simulink model "three_level_ttype_pwm"  (R2025a)
settings: Solver=ode1be  StartTime=0.0  StopTime=simlength  FixedStep=ts_sim  MaxStep=ts_sim
undefined symbols (not defined in the file): fPWM_INV, kp_dudc, number_of_cells, Q, q1Kalman, q2Kalman, q3Kalman, rKalman, tc, ts_zvs, tsample, Vbattery_nom
libraries: fl_lib x54, nesl_utility x31, lithium_ion_cell_lib x1, simulink x1
(part 1 of 2)
settings Model: SimulationMode=accelerator  Creator=LTNBDA  LastModifiedBy=ltnbda
settings SolverCC: ZeroCrossControl=EnableAll  ZeroCrossAlgorithm=Adaptive  AlgebraicLoopSolver=TrustRegion  SolverResetMethod=Robust  AutoInsertRateTranBlk=on
settings DataIOCC: LimitDataPoints=on  MaxDataPoints=1  SaveFormat=Array  SignalLoggingSaveFormat=ModelDataLogs  SaveOutput=off  SignalLogging=off  DSMLogging=off  SaveTime=off  ReturnWorkspaceOutputs=off
settings OptimizationCC: ExpressionDepthLimit=2147483647.0  InitFltsAndDblsToZero=on  EfficientMapNaN2IntZero=off  LifeSpan=inf
settings DebuggingCC: SaveWithParameterizedLinksMsg=none  UnderspecifiedInitializationDetection=Classic  MergeDetectMultiDrivingBlocksExec=none  SignalResolutionControl=TryResolveAllWithWarning  SolverPrmCheckMsg=warning  MultiTaskDSMMsg=warning  MultiTaskCondExecSysMsg=none  MultiTaskRateTransMsg=warning  FcnCallInpInsideContextMsg=warning  StateNameClashWarn=warning  SFUnexpectedBacktrackingDiag=warning  SFNoUnconditionalDefaultTransitionDiag=warning  ArithmeticOperatorsInVariantConditions=warning
settings HardwareCC: ProdBitPerLong=64.0  ProdLargestAtomicFloat=None  ProdIntDivRoundTo=Undefined  ProdEndianess=Unspecified  ProdHWDeviceType=Generic->64-bit Embedded Processor (LP64)  TargetBitPerPointer=64.0  TargetBitPerSizeT=64.0  TargetBitPerPtrDiffT=64.0  TargetLongLongMode=on  TargetIntDivRoundTo=Zero  TargetEndianess=LittleEndian  TargetWordSize=64.0  TargetHWDeviceType=MATLAB Host  ProdEqTarget=off
settings ModelReferenceCC: EnableRefExpFcnMdlSchedulingChecks=on  PropagateSignalLabelsOutOfModel=off
settings SFSimCC: SimUseLocalCustomCode=off  CustomCodeUndefinedFunction=UseInterfaceOnly
settings RTWCC: RTWUseLocalCustomCode=off  GPUComputeCapability=3.5
settings CodeAppCC: MaxIdLength=128.0  StateflowObjectComments=on
settings GRTTargetCC: TargetLangStandard=C89/C90 (ANSI)  CombineOutputUpdateFcns=off  GRTInterface=on
settings ConfigComp: CovMetricSettings=dw  CovSaveCumulativeToWorkspaceVar=on  CovSaveSingleToWorkspaceVar=on  CovExternalEMLEnable=off
settings SimscapeCC: SimscapeNormalizeSystem=off

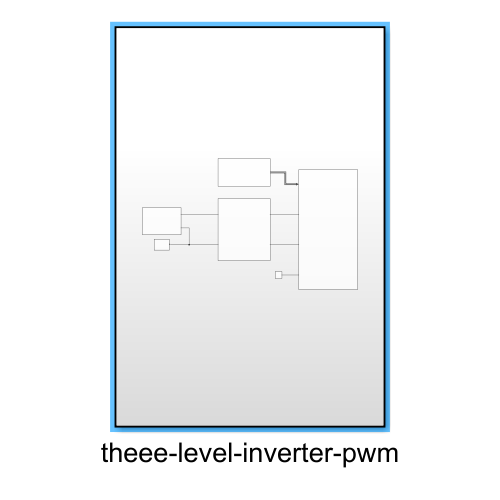
[thumbnail: Simulink's stored preview of the top-level diagram]
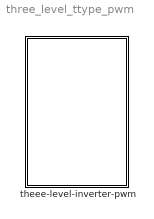
== system three_level_ttype_pwm ==
  theee-level-inverter-pwm : Subsystem

== system three_level_ttype_pwm/theee-level-inverter-pwm ==
  Electrical Reference2 : fl_lib/Electrical/Electrical Elements/Electrical Reference
  Solver Configuration : nesl_utility/Solver Configuration  PhysicalDomain=network_engine_domain  SubClassName=solver  LeftPortType=input  RightPortType=generic  Tones=[]  Harmonics=[]  SimulateNoise=off  Profile=off  UseLocalSampling=off  EnableSwitchedLinearOptims=on  FrequencyDomain=off  UseCCode=off  RelTol=0.001  AbsTol=0.001  MinStep=1e-09  ToWorkspace=off  RevertToSquareIcSolve=off  NumHomotopyIterations=100  PhasorMode=off  PhasorModeNumHarmonics=1  ConsistencySolver=NEWTON_FTOL  IndexReductionMethod=DerivativeReplacement  DoDC=on  ResidualTolerance=1e-09  ConsistencyTolSource=GLOBAL  ConsistencyAbsTol=0.001  ConsistencyRelTol=0.001  ConsistencyTolFactor=0.001  UseLocalSolver=on  LocalSolverChoice=NE_BACKWARD_EULER_ADVANCER  ResolveIndetEquations=on  FunctionEvalNumThread=1  LocalSolverSampleTime=ts_sim  DoFixedCost=off  MaxNonlinIter=3  MaxModeIter=2  ComputeImpulses=off  ImpulseIterations=2  LinearAlgebra=auto  LinearAlgebraNumThread=0  EquationFormulation=NE_TIME_EF  DelaysMemoryBudget=1024  AutomaticFiltering=on  FilteringTimeConstant=0.001  PartitionStorageMethod=AS_NEEDED  PartitionMemoryBudget=1024  PartitionMethod=ROBUST  MultibodyUseLocalSolver=off  MultibodyLocalSolverChoice=ODE1  MultibodyLocalSolverSampleTime=0.001
  battery_system : Subsystem
  pwm_commands : Subsystem
  single_phase_ui_measure1 : Subsystem
  three-level-inverter : Subsystem
  wires:
  pwm_commands/1(gate_commands) -> three-level-inverter/1(gate_commands)
  connections:
  single_phase_ui_measure1/LConn2 -- Solver Configuration/RConn1 -- battery_system/RConn2
  single_phase_ui_measure1/RConn1 -- three-level-inverter/LConn1
  battery_system/RConn1 -- single_phase_ui_measure1/LConn1
  three-level-inverter/LConn2 -- single_phase_ui_measure1/RConn2
  Electrical Reference2/LConn1 -- three-level-inverter/LConn3

== system three_level_ttype_pwm/theee-level-inverter-pwm/battery_system ==
  LithiumIonBattery : Subsystem
  Uout+ : PMIOPort  Side=Right
  Uout- : PMIOPort  Port=2  Side=Right
  connections:
  LithiumIonBattery/RConn1 -- Uout+/RConn1
  LithiumIonBattery/RConn2 -- Uout-/RConn1

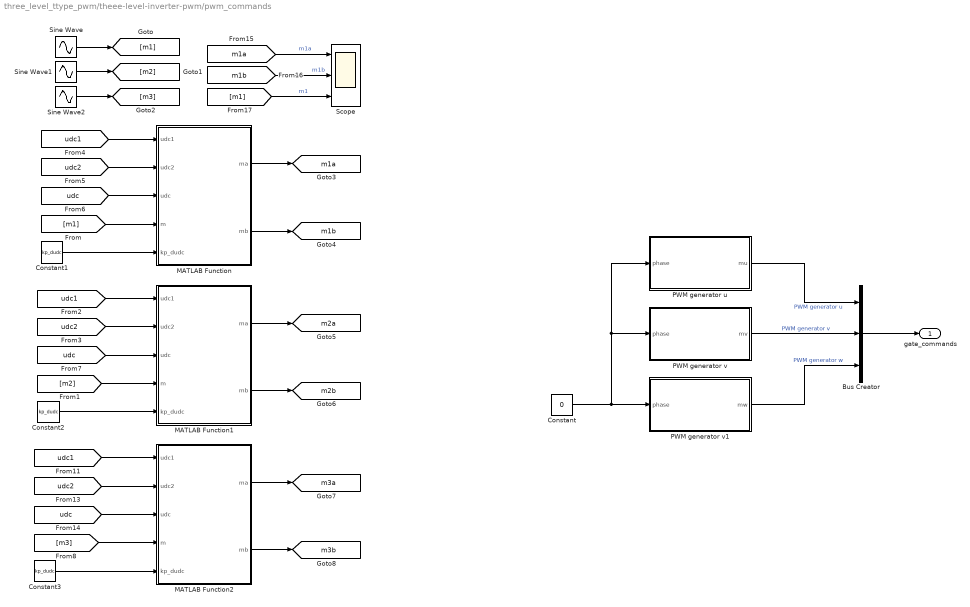
== system three_level_ttype_pwm/theee-level-inverter-pwm/pwm_commands ==
  Bus Creator : BusCreator  Inputs=3
  Constant : Constant  Value=0
  Constant1 : Constant  Value=kp_dudc
  Constant2 : Constant  Value=kp_dudc
  Constant3 : Constant  Value=kp_dudc
  MATLAB Function : MATLAB Function  TreatAsAtomicUnit=on
  MATLAB Function1 : MATLAB Function  TreatAsAtomicUnit=on
  MATLAB Function2 : MATLAB Function  TreatAsAtomicUnit=on
  PWM generator u : Subsystem  mask{f=fPWM_INV, m_up=1, m_low=-1, dead_time=0, pos_cmd_gate=1, neg_cmd_gate=0, polarity=1}
      mask prompts: f "Frequency (Hz)"; m_up "Max Input Modulation Value"; m_low "Min Input Modulation Value"; dead_time "Dead Time (s)"; pos_cmd_gate "Positive Gate Voltage (V)"; neg_cmd_gate "Negative Gate Voltage (V)"; polarity "Polarity (pu)"
  PWM generator v : Subsystem  mask{f=fPWM_INV, m_up=1, m_low=-1, dead_time=0, pos_cmd_gate=1, neg_cmd_gate=0, polarity=1}
      mask prompts: f "Frequency (Hz)"; m_up "Max Input Modulation Value"; m_low "Min Input Modulation Value"; dead_time "Dead Time (s)"; pos_cmd_gate "Positive Gate Voltage (V)"; neg_cmd_gate "Negative Gate Voltage (V)"; polarity "Polarity (pu)"
  PWM generator v1 : Subsystem  mask{f=fPWM_INV, m_up=1, m_low=-1, dead_time=0, pos_cmd_gate=1, neg_cmd_gate=0, polarity=1}
      mask prompts: f "Frequency (Hz)"; m_up "Max Input Modulation Value"; m_low "Min Input Modulation Value"; dead_time "Dead Time (s)"; pos_cmd_gate "Positive Gate Voltage (V)"; neg_cmd_gate "Negative Gate Voltage (V)"; polarity "Polarity (pu)"
  Scope : Scope  NumInputPorts=3
      settings: ActiveDisplayYMinimum=-1.0203710782461322  ActiveDisplayYMaximum=1.0167997732254843
  Sine Wave : Sin  Amplitude=0.8  Frequency=2*pi*50  SampleTime=0
  Sine Wave1 : Sin  Amplitude=0.8  Frequency=2*pi*50  Phase=-2*pi/3  SampleTime=0
  Sine Wave2 : Sin  Amplitude=0.8  Frequency=2*pi*50  Phase=2*pi/3  SampleTime=0
  gate_commands : Outport
  tag scope: m1a=global, m1b=global, m2a=global, m2b=global, m3a=global, m3b=global
  wires:
  PWM generator v/1(mv) -> Bus Creator/2  "PWM generator v"
  PWM generator u/1(mu) -> Bus Creator/1  "PWM generator u"
  PWM generator v1/1(mw) -> Bus Creator/3  "PWM generator w"
  Constant/1 -> PWM generator u/1(phase), PWM generator v/1(phase), PWM generator v1/1(phase)
  Sine Wave/1 -> [m1]
  Sine Wave1/1 -> [m2]
  Sine Wave2/1 -> [m3]
  [m1] -> MATLAB Function/4(m)
  MATLAB Function/1(ma) -> [m1a]
  MATLAB Function/2(mb) -> [m1b]
  MATLAB Function1/1(ma) -> [m2a]
  MATLAB Function1/2(mb) -> [m2b]
  [m2] -> MATLAB Function1/4(m)
  MATLAB Function2/1(ma) -> [m3a]
  MATLAB Function2/2(mb) -> [m3b]
  [m1a] -> Scope/1  "m1a"
  [m1b] -> Scope/2  "m1b"
  [m3] -> MATLAB Function2/4(m)
  [udc] -> MATLAB Function/3(udc)
  [udc] -> MATLAB Function1/3(udc)
  [m1] -> Scope/3  "m1"
  [udc] -> MATLAB Function2/3(udc)
  Constant1/1 -> MATLAB Function/5(kp_dudc)
  Constant2/1 -> MATLAB Function1/5(kp_dudc)
  Constant3/1 -> MATLAB Function2/5(kp_dudc)
  [udc1] -> MATLAB Function/1(udc1)
  [udc2] -> MATLAB Function/2(udc2)
  [udc1] -> MATLAB Function1/1(udc1)
  [udc2] -> MATLAB Function1/2(udc2)
  [udc1] -> MATLAB Function2/1(udc1)
  [udc2] -> MATLAB Function2/2(udc2)
  Bus Creator/1 -> gate_commands/1

== system three_level_ttype_pwm/theee-level-inverter-pwm/single_phase_ui_measure1 ==
  Bus Creator : BusCreator  Inputs=2
  Current Sensor : fl_lib/Electrical/Electrical Sensors/Current Sensor
  Selector : Selector  InputPortWidth=2  IndexOptions=Index vector (dialog)  Indices=2  OutputSizes=1
  Selector1 : Selector  InputPortWidth=2  IndexOptions=Index vector (dialog)  Indices=1  OutputSizes=1
  Transfer Fcn : TransferFcn  Denominator=[1e-4 1]
  Voltage Sensor : fl_lib/Electrical/Electrical Sensors/Voltage Sensor
  input : Scope  NumInputPorts=2
      settings: SampleTime=tc  ActiveDisplayYMinimum=-52.828591960664284  ActiveDisplayYMaximum=475.45762649280624  DataLoggingVariableName=ScopeData2
  iph : nesl_utility/PS-Simulink Converter  PhysicalDomain=network_engine_domain  SubClassName=ps_output  LeftPortType=input  RightPortType=output  PseudoPeriodic=off  Frequencies=[]  VectorFormat=1-D array  Unit=A  AffineConversion=off
  uph : nesl_utility/PS-Simulink Converter  PhysicalDomain=network_engine_domain  SubClassName=ps_output  LeftPortType=input  RightPortType=output  PseudoPeriodic=off  Frequencies=[]  VectorFormat=1-D array  Unit=V  AffineConversion=off
  Udc(+) : PMIOPort  Side=Left
  udc(+) : PMIOPort  Port=2  Side=Right
  Udc(-) : PMIOPort  Port=3  Side=Left
  udc(-) : PMIOPort  Port=4  Side=Right
  tag scope: current_battery=global, voltage_battery=global
  wires:
  Selector/1 -> input/2, [voltage_battery]  "voltage_battery"
  Selector1/1 -> input/1, Transfer Fcn/1  "current_battery"
  uph/1 -> Bus Creator/2  "uph"
  iph/1 -> Bus Creator/1  "iph"
  Bus Creator/1 -> Selector1/1, Selector/1  "ui_data"
  Transfer Fcn/1 -> [current_battery]
  connections:
  udc(-)/RConn1 -- Udc(-)/RConn1 -- Voltage Sensor/RConn2
  Voltage Sensor/RConn1 -- uph/LConn1
  Current Sensor/RConn2 -- udc(+)/RConn1
  Udc(+)/RConn1 -- Current Sensor/LConn1 -- Voltage Sensor/LConn1
  iph/LConn1 -- Current Sensor/RConn1

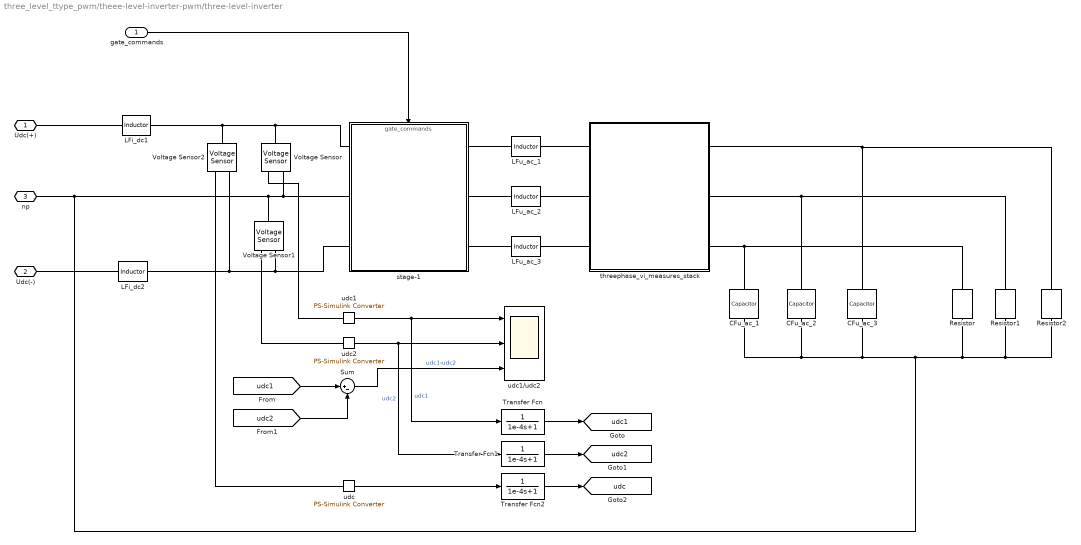
== system three_level_ttype_pwm/theee-level-inverter-pwm/three-level-inverter ==
  gate_commands : Inport
  CFu_ac_1 : fl_lib/Electrical/Electrical Elements/Capacitor  c=400e-6 F  r=5e-3 Ohm  g=0 1/Ohm  i_specify=off  i_priority=None  i=0 A  i_nominal_specify=off  i_nominal_value=1  i_nominal_unit=A  v_specify=off  v_priority=None  v=0 V  v_nominal_specify=off  v_nominal_value=1  v_nominal_unit=V  vc_specify=off  vc_priority=High  vc=0 V  vc_nominal_specify=off  vc_nominal_value=1  vc_nominal_unit=V
  CFu_ac_2 : fl_lib/Electrical/Electrical Elements/Capacitor  c=400e-6 F  r=5e-3 Ohm  g=0 1/Ohm  i_specify=off  i_priority=None  i=0 A  i_nominal_specify=off  i_nominal_value=1  i_nominal_unit=A  v_specify=off  v_priority=None  v=0 V  v_nominal_specify=off  v_nominal_value=1  v_nominal_unit=V  vc_specify=off  vc_priority=High  vc=0 V  vc_nominal_specify=off  vc_nominal_value=1  vc_nominal_unit=V
  CFu_ac_3 : fl_lib/Electrical/Electrical Elements/Capacitor  c=400e-6 F  r=5e-3 Ohm  g=0 1/Ohm  i_specify=off  i_priority=None  i=0 A  i_nominal_specify=off  i_nominal_value=1  i_nominal_unit=A  v_specify=off  v_priority=None  v=0 V  v_nominal_specify=off  v_nominal_value=1  v_nominal_unit=V  vc_specify=off  vc_priority=High  vc=0 V  vc_nominal_specify=off  vc_nominal_value=1  vc_nominal_unit=V
  LFi_dc1 : fl_lib/Electrical/Electrical Elements/Inductor  l=Ldc1 H  r=RLdc1 Ohm  g=1e-9 1/Ohm  i_specify=on  i_priority=High  i=0 A  i_nominal_specify=off  i_nominal_value=1  i_nominal_unit=A  v_specify=off  v_priority=None  v=0 V  v_nominal_specify=off  v_nominal_value=1  v_nominal_unit=V  i_L_specify=off  i_L_priority=High  i_L=0 A  i_L_nominal_specify=off  i_L_nominal_value=1  i_L_nominal_unit=A
  LFi_dc2 : fl_lib/Electrical/Electrical Elements/Inductor  l=Ldc2 H  r=Ldc2 Ohm  g=1e-9 1/Ohm  i_specify=on  i_priority=High  i=0 A  i_nominal_specify=off  i_nominal_value=1  i_nominal_unit=A  v_specify=off  v_priority=None  v=0 V  v_nominal_specify=off  v_nominal_value=1  v_nominal_unit=V  i_L_specify=off  i_L_priority=High  i_L=0 A  i_L_nominal_specify=off  i_L_nominal_value=1  i_L_nominal_unit=A
  LFu_ac_1 : fl_lib/Electrical/Electrical Elements/Inductor  l=250e-6 H  r=3e-3 Ohm  g=1e-9 1/Ohm  i_specify=off  i_priority=None  i=0 A  i_nominal_specify=off  i_nominal_value=1  i_nominal_unit=A  v_specify=off  v_priority=None  v=0 V  v_nominal_specify=off  v_nominal_value=1  v_nominal_unit=V  i_L_specify=off  i_L_priority=High  i_L=0 A  i_L_nominal_specify=off  i_L_nominal_value=1  i_L_nominal_unit=A
  LFu_ac_2 : fl_lib/Electrical/Electrical Elements/Inductor  l=250e-6 H  r=3e-3 Ohm  g=1e-9 1/Ohm  i_specify=off  i_priority=None  i=0 A  i_nominal_specify=off  i_nominal_value=1  i_nominal_unit=A  v_specify=off  v_priority=None  v=0 V  v_nominal_specify=off  v_nominal_value=1  v_nominal_unit=V  i_L_specify=off  i_L_priority=High  i_L=0 A  i_L_nominal_specify=off  i_L_nominal_value=1  i_L_nominal_unit=A
  LFu_ac_3 : fl_lib/Electrical/Electrical Elements/Inductor  l=250e-6 H  r=3e-3 Ohm  g=1e-9 1/Ohm  i_specify=off  i_priority=None  i=0 A  i_nominal_specify=off  i_nominal_value=1  i_nominal_unit=A  v_specify=off  v_priority=None  v=0 V  v_nominal_specify=off  v_nominal_value=1  v_nominal_unit=V  i_L_specify=off  i_L_priority=High  i_L=0 A  i_L_nominal_specify=off  i_L_nominal_value=1  i_L_nominal_unit=A
  Resistor : fl_lib/Electrical/Electrical Elements/Resistor  R=1.6 Ohm  i_specify=off  i_priority=None  i=0 A  i_nominal_specify=off  i_nominal_value=1  i_nominal_unit=A  v_specify=off  v_priority=None  v=0 V  v_nominal_specify=off  v_nominal_value=1  v_nominal_unit=V
  Resistor1 : fl_lib/Electrical/Electrical Elements/Resistor  R=1.6 Ohm  i_specify=off  i_priority=None  i=0 A  i_nominal_specify=off  i_nominal_value=1  i_nominal_unit=A  v_specify=off  v_priority=None  v=0 V  v_nominal_specify=off  v_nominal_value=1  v_nominal_unit=V
  Resistor2 : fl_lib/Electrical/Electrical Elements/Resistor  R=1.6 Ohm  i_specify=off  i_priority=None  i=0 A  i_nominal_specify=off  i_nominal_value=1  i_nominal_unit=A  v_specify=off  v_priority=None  v=0 V  v_nominal_specify=off  v_nominal_value=1  v_nominal_unit=V
  Sum : Sum  Inputs=|+-
  Transfer Fcn : TransferFcn  Denominator=[1e-4 1]
  Transfer Fcn1 : TransferFcn  Denominator=[1e-4 1]
  Transfer Fcn2 : TransferFcn  Denominator=[1e-4 1]
  Voltage Sensor : fl_lib/Electrical/Electrical Sensors/Voltage Sensor
  Voltage Sensor1 : fl_lib/Electrical/Electrical Sensors/Voltage Sensor
  Voltage Sensor2 : fl_lib/Electrical/Electrical Sensors/Voltage Sensor
  stage-1 : Subsystem
      settings: PortSchema="{\"entries\":[{\"content\":{\"sides\":[{\"content\":{\"connectorIds\":[\"LConn1\",\"LConn2\",\"LConn3\"]},\"type\":\"ConnectorPlacement.EquallySpacedRectSide\",\"uuid\":\"c872503a-61af-4937-bdf2-4de4f8645573\"},{\"content\":{\"connectorIds\":[\"RConn1\",\"RConn2\",\"RConn3\"],\"side\":\"RIGHT\"},\"type\":\"ConnectorPlacement.EquallySpacedRectSide\",\"uuid\":\"3b83f060-86a2-4569-84b5-d9f7c0485347\"},{\"content\":{\"connectorIds\":[\"In1\"],\"side\":\"TOP\"},\"type\":\"ConnectorPlacement.EquallySpacedRectSide\",\"uuid\":\"bf191d46-ce71-4d15-9dd0-24cc57253577\"}]},\"type\":\"ConnectorPlacement.EquallySpacedConnector\",\"uuid\":\"1b28ceee-25d0-45ae-a3c4-c2563f0d63ba\"}],\"packageUris\":[\"http://schema.mathworks.com/mf0/Connector/R2020b\"],\"version\":\"1.0\"}"
  threephase_vi_measures_stack : Subsystem
  udc : nesl_utility/PS-Simulink Converter  PhysicalDomain=network_engine_domain  SubClassName=ps_output  LeftPortType=input  RightPortType=output  PseudoPeriodic=off  Frequencies=[]  VectorFormat=1-D array  Unit=V  AffineConversion=off
  udc1 : nesl_utility/PS-Simulink Converter  PhysicalDomain=network_engine_domain  SubClassName=ps_output  LeftPortType=input  RightPortType=output  PseudoPeriodic=off  Frequencies=[]  VectorFormat=1-D array  Unit=V  AffineConversion=off
  udc1/udc2 : Scope  NumInputPorts=3
      settings: SampleTime=tc  ActiveDisplayYMinimum=459.3584684150768  ActiveDisplayYMaximum=553.49695314359838  DataLoggingVariableName=ScopeData5
  udc2 : nesl_utility/PS-Simulink Converter  PhysicalDomain=network_engine_domain  SubClassName=ps_output  LeftPortType=input  RightPortType=output  PseudoPeriodic=off  Frequencies=[]  VectorFormat=1-D array  Unit=V  AffineConversion=off
  Udc(+) : PMIOPort  Side=Left
  Udc(-) : PMIOPort  Port=2  Side=Left
  np : PMIOPort  Port=3  Side=Left
  tag scope: udc1=global, udc2=global, udc=global
  wires:
  udc2/1 -> Transfer Fcn1/1, udc1/udc2/2  "udc2"
  udc1/1 -> Transfer Fcn/1, udc1/udc2/1  "udc1"
  gate_commands/1 -> stage-1/1(gate_commands)
  udc/1 -> Transfer Fcn2/1
  Transfer Fcn/1 -> [udc1]
  Transfer Fcn1/1 -> [udc2]
  Transfer Fcn2/1 -> [udc]
  [udc1] -> Sum/1
  [udc2] -> Sum/2
  Sum/1 -> udc1/udc2/3  "udc1-udc2"
  connections:
  LFi_dc2/RConn1 -- Voltage Sensor2/RConn2 -- stage-1/RConn3 -- Voltage Sensor1/RConn2
  Voltage Sensor/RConn1 -- udc1/LConn1
  Voltage Sensor1/RConn1 -- udc2/LConn1
  CFu_ac_3/LConn1 -- Resistor2/LConn1 -- threephase_vi_measures_stack/RConn1
  CFu_ac_2/LConn1 -- Resistor1/LConn1 -- threephase_vi_measures_stack/RConn2
  threephase_vi_measures_stack/RConn3 -- Resistor/LConn1 -- CFu_ac_1/LConn1
  LFu_ac_3/RConn1 -- threephase_vi_measures_stack/LConn3
  LFu_ac_2/RConn1 -- threephase_vi_measures_stack/LConn2
  LFu_ac_1/RConn1 -- threephase_vi_measures_stack/LConn1
  stage-1/LConn3 -- LFu_ac_3/LConn1
  stage-1/LConn1 -- LFu_ac_1/LConn1
  LFu_ac_2/LConn1 -- stage-1/LConn2
  Voltage Sensor/LConn1 -- LFi_dc1/RConn1 -- Voltage Sensor2/LConn1 -- stage-1/RConn1
  LFi_dc1/LConn1 -- Udc(+)/RConn1
  Voltage Sensor2/RConn1 -- udc/LConn1
  Udc(-)/RConn1 -- LFi_dc2/LConn1
  Voltage Sensor/RConn2 -- np/RConn1 -- Resistor1/RConn1 -- Resistor2/RConn1 -- Resistor/RConn1 -- CFu_ac_2/RConn1 -- CFu_ac_1/RConn1 -- CFu_ac_3/RConn1 -- Voltage Sensor1/LConn1 -- stage-1/RConn2

== system three_level_ttype_pwm/theee-level-inverter-pwm/battery_system/LithiumIonBattery ==
  Current Sensor : fl_lib/Electrical/Electrical Sensors/Current Sensor
  PS-Simulink Converter4 : nesl_utility/PS-Simulink Converter  PhysicalDomain=network_engine_domain  SubClassName=ps_output  LeftPortType=input  RightPortType=output  PseudoPeriodic=off  Frequencies=[]  VectorFormat=1-D array  Unit=1  AffineConversion=off
  PS-Simulink Converter5 : nesl_utility/PS-Simulink Converter  PhysicalDomain=network_engine_domain  SubClassName=ps_output  LeftPortType=input  RightPortType=output  PseudoPeriodic=off  Frequencies=[]  VectorFormat=1-D array  Unit=V  AffineConversion=on
  SOC_estimator : Subsystem  Commented=on
  To Workspace1 : ToWorkspace  VariableName=idc_battery_sim  SampleTime=tc
      settings: MaxDataPoints=Nc
  To Workspace2 : ToWorkspace  VariableName=udc_battery_sim  SampleTime=tc
      settings: MaxDataPoints=Nc
  Unit Delay5 : UnitDelay  SampleTime=ts_zvs  HasFrameUpgradeWarning=on
  Voltage Sensor : fl_lib/Electrical/Electrical Sensors/Voltage Sensor
  ibat/vdc : Scope  NumInputPorts=2
      settings: SampleTime=tc  ActiveDisplayYMinimum=-124.51886598951859  ActiveDisplayYMaximum=1120.6697939056676  DataLoggingVariableName=ScopeData6
  lithium ion cell analytical ocv : Subsystem
  Uout+ : PMIOPort  Side=Right
  Uout- : PMIOPort  Port=2  Side=Right
  wires:
  [vdc] -> ibat/vdc/2  "vdc"
  Unit Delay5/1 -> [vdc], To Workspace2/1
  PS-Simulink Converter4/1 -> ibat/vdc/1, To Workspace1/1  "i batt"
  PS-Simulink Converter5/1 -> Unit Delay5/1
  connections:
  lithium ion cell analytical ocv/RConn1 -- Current Sensor/LConn1
  Uout-/RConn1 -- lithium ion cell analytical ocv/RConn2 -- Voltage Sensor/RConn2
  Voltage Sensor/RConn1 -- PS-Simulink Converter5/LConn1
  Voltage Sensor/LConn1 -- Current Sensor/RConn2 -- Uout+/RConn1
  Current Sensor/RConn1 -- PS-Simulink Converter4/LConn1

== system three_level_ttype_pwm/theee-level-inverter-pwm/pwm_commands/PWM generator u ==
  phase : Inport
  Bus Creator : BusCreator  Inputs=4
  carry_n : Subsystem
  carry_p : Subsystem
  modulator_n : Subsystem
  modulator_p : Subsystem
  mu : Outport
  wires:
  phase/1 -> carry_n/1(phase), carry_p/1(phase)
  carry_p/1(trp) -> modulator_p/1(tr)  "trp"
  carry_n/1(trn) -> modulator_n/1(tr)  "trn"
  modulator_p/1(m1) -> [m1]
  modulator_p/2(m3) -> [m3]
  modulator_n/1(m2) -> [m2]
  modulator_n/2(m4) -> [m4]
  [m1] -> Bus Creator/1  "m1u"
  [m2] -> Bus Creator/2  "m2u"
  [m3] -> Bus Creator/3  "m3u"
  [m4] -> Bus Creator/4  "m4u"
  Bus Creator/1 -> mu/1  "p"
  [m1a] -> modulator_p/2(m_index)
  [m1b] -> modulator_n/2(m_index)

== system three_level_ttype_pwm/theee-level-inverter-pwm/pwm_commands/PWM generator v ==
  phase : Inport
  Bus Creator : BusCreator  Inputs=4
  carry_n : Subsystem
  carry_p : Subsystem
  modulator_n : Subsystem
  modulator_p : Subsystem
  mv : Outport
  wires:
  [m2b] -> modulator_n/2(m_index)
  [m2a] -> modulator_p/2(m_index)
  Bus Creator/1 -> mv/1  "p"
  [m4] -> Bus Creator/4  "m4v"
  [m3] -> Bus Creator/3  "m3v"
  [m2] -> Bus Creator/2  "m2v"
  [m1] -> Bus Creator/1  "m1v"
  modulator_n/2(m4) -> [m4]
  modulator_n/1(m2) -> [m2]
  modulator_p/2(m3) -> [m3]
  modulator_p/1(m1) -> [m1]
  carry_n/1(trn) -> modulator_n/1(tr)  "trn"
  carry_p/1(trp) -> modulator_p/1(tr)  "trp"
  phase/1 -> carry_p/1(phase), carry_n/1(phase)

== system three_level_ttype_pwm/theee-level-inverter-pwm/pwm_commands/PWM generator v1 ==
  phase : Inport
  Bus Creator : BusCreator  Inputs=4
  carry_n : Subsystem
  carry_p : Subsystem
  modulator_n : Subsystem
  modulator_p : Subsystem
  mw : Outport
  wires:
  phase/1 -> carry_n/1(phase), carry_p/1(phase)
  carry_p/1(trp) -> modulator_p/1(tr)  "trp"
  carry_n/1(trn) -> modulator_n/1(tr)  "trn"
  modulator_p/1(m1) -> [m1]
  modulator_p/2(m3) -> [m3]
  modulator_n/1(m2) -> [m2]
  modulator_n/2(m4) -> [m4]
  [m1] -> Bus Creator/1  "m1w"
  [m2] -> Bus Creator/2  "m2w"
  [m3] -> Bus Creator/3  "m3w"
  [m4] -> Bus Creator/4  "m4w"
  Bus Creator/1 -> mw/1  "p"
  [m3a] -> modulator_p/2(m_index)
  [m3b] -> modulator_n/2(m_index)

== system three_level_ttype_pwm/theee-level-inverter-pwm/three-level-inverter/stage-1 ==
  gate_commands : Inport
  Cdc1 : fl_lib/Electrical/Electrical Elements/Capacitor  c=Cdc1 F  r=RCdc1 Ohm  g=0 1/Ohm  i_specify=off  i_priority=None  i=0 A  i_nominal_specify=off  i_nominal_value=1  i_nominal_unit=A  v_specify=off  v_priority=High  v=Vbattery_nom/2 V  v_nominal_specify=off  v_nominal_value=1  v_nominal_unit=V  vc_specify=on  vc_priority=High  vc=Vbattery_nom/2 V  vc_nominal_specify=off  vc_nominal_value=1  vc_nominal_unit=V
  Cdc2 : fl_lib/Electrical/Electrical Elements/Capacitor  c=Cdc2 F  r=RCdc2 Ohm  g=0 1/Ohm  i_specify=off  i_priority=None  i=0 A  i_nominal_specify=off  i_nominal_value=1  i_nominal_unit=A  v_specify=off  v_priority=High  v=Vbattery_nom/2 V  v_nominal_specify=off  v_nominal_value=1  v_nominal_unit=V  vc_specify=on  vc_priority=High  vc=Vbattery_nom/2 V  vc_nominal_specify=off  vc_nominal_value=1  vc_nominal_unit=V
  three-level-inverter2 : Subsystem
  uu : PMIOPort  Side=Left
  uv : PMIOPort  Port=2  Side=Left
  Udc(+) : PMIOPort  Port=3  Side=Right
  np : PMIOPort  Port=4  Side=Right
  Udc(-) : PMIOPort  Port=5  Side=Right
  uw : PMIOPort  Port=6  Side=Left
  wires:
  gate_commands/1 -> three-level-inverter2/1(gate_commands)
  connections:
  Cdc2/LConn1 -- three-level-inverter2/RConn2 -- np/RConn1 -- Cdc1/RConn1
  Cdc2/RConn1 -- three-level-inverter2/RConn3 -- Udc(-)/RConn1
  three-level-inverter2/LConn3 -- uw/RConn1
  Udc(+)/RConn1 -- three-level-inverter2/RConn1 -- Cdc1/LConn1
  three-level-inverter2/LConn2 -- uv/RConn1
  three-level-inverter2/LConn1 -- uu/RConn1

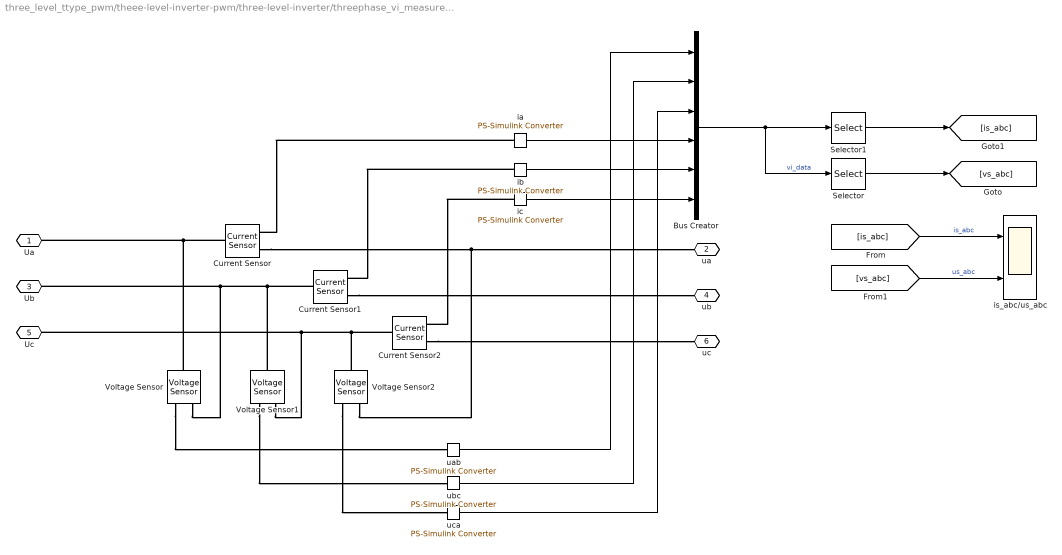
== system three_level_ttype_pwm/theee-level-inverter-pwm/three-level-inverter/threephase_vi_measures_stack ==
  Bus Creator : BusCreator  Inputs=6
  Current Sensor : fl_lib/Electrical/Electrical Sensors/Current Sensor
  Current Sensor1 : fl_lib/Electrical/Electrical Sensors/Current Sensor
  Current Sensor2 : fl_lib/Electrical/Electrical Sensors/Current Sensor
  Selector : Selector  InputPortWidth=6  IndexOptions=Index vector (dialog)  Indices=[1 2 3]  OutputSizes=1
  Selector1 : Selector  InputPortWidth=6  IndexOptions=Index vector (dialog)  Indices=[4 5 6]  OutputSizes=1
  Voltage Sensor : fl_lib/Electrical/Electrical Sensors/Voltage Sensor
  Voltage Sensor1 : fl_lib/Electrical/Electrical Sensors/Voltage Sensor
  Voltage Sensor2 : fl_lib/Electrical/Electrical Sensors/Voltage Sensor
  ia : nesl_utility/PS-Simulink Converter  PhysicalDomain=network_engine_domain  SubClassName=ps_output  LeftPortType=input  RightPortType=output  PseudoPeriodic=off  Frequencies=[]  VectorFormat=1-D array  Unit=A  AffineConversion=off
  ib : nesl_utility/PS-Simulink Converter  PhysicalDomain=network_engine_domain  SubClassName=ps_output  LeftPortType=input  RightPortType=output  PseudoPeriodic=off  Frequencies=[]  VectorFormat=1-D array  Unit=A  AffineConversion=off
  ic : nesl_utility/PS-Simulink Converter  PhysicalDomain=network_engine_domain  SubClassName=ps_output  LeftPortType=input  RightPortType=output  PseudoPeriodic=off  Frequencies=[]  VectorFormat=1-D array  Unit=A  AffineConversion=off
  is_abc/us_abc : Scope  NumInputPorts=2
      settings: SampleTime=tc  ActiveDisplayYMinimum=-668.55946592135967  ActiveDisplayYMaximum=605.99408770505715
  uab : nesl_utility/PS-Simulink Converter  PhysicalDomain=network_engine_domain  SubClassName=ps_output  LeftPortType=input  RightPortType=output  PseudoPeriodic=off  Frequencies=[]  VectorFormat=1-D array  Unit=V  AffineConversion=off
  ubc : nesl_utility/PS-Simulink Converter  PhysicalDomain=network_engine_domain  SubClassName=ps_output  LeftPortType=input  RightPortType=output  PseudoPeriodic=off  Frequencies=[]  VectorFormat=1-D array  Unit=V  AffineConversion=off
  uca : nesl_utility/PS-Simulink Converter  PhysicalDomain=network_engine_domain  SubClassName=ps_output  LeftPortType=input  RightPortType=output  PseudoPeriodic=off  Frequencies=[]  VectorFormat=1-D array  Unit=V  AffineConversion=off
  Ua : PMIOPort  Side=Left
  ua : PMIOPort  Port=2  Side=Right
  Ub : PMIOPort  Port=3  Side=Left
  ub : PMIOPort  Port=4  Side=Right
  Uc : PMIOPort  Port=5  Side=Left
  uc : PMIOPort  Port=6  Side=Right
  wires:
  uca/1 -> Bus Creator/3
  ubc/1 -> Bus Creator/2
  uab/1 -> Bus Creator/1
  [vs_abc] -> is_abc/us_abc/2  "us_abc"
  [is_abc] -> is_abc/us_abc/1  "is_abc"
  Selector1/1 -> [is_abc]
  ic/1 -> Bus Creator/6
  ia/1 -> Bus Creator/4
  ib/1 -> Bus Creator/5
  Selector/1 -> [vs_abc]
  Bus Creator/1 -> Selector1/1, Selector/1  "vi_data"
  connections:
  Current Sensor2/RConn2 -- uc/RConn1
  ic/LConn1 -- Current Sensor2/RConn1
  ia/LConn1 -- Current Sensor/RConn1
  ib/LConn1 -- Current Sensor1/RConn1
  Voltage Sensor2/RConn1 -- uca/LConn1
  Current Sensor1/RConn2 -- ub/RConn1
  Voltage Sensor/LConn1 -- Current Sensor/LConn1 -- Ua/RConn1
  Current Sensor2/LConn1 -- Voltage Sensor2/LConn1 -- Voltage Sensor1/RConn2 -- Uc/RConn1
  Voltage Sensor1/RConn1 -- ubc/LConn1
  Voltage Sensor2/RConn2 -- Current Sensor/RConn2 -- ua/RConn1
  Voltage Sensor/RConn1 -- uab/LConn1
  Voltage Sensor1/LConn1 -- Current Sensor1/LConn1 -- Voltage Sensor/RConn2 -- Ub/RConn1

== system three_level_ttype_pwm/theee-level-inverter-pwm/battery_system/LithiumIonBattery/SOC_estimator ==
  Kalman_observer : Subsystem
  SOC*/SOC : Scope  Commented=on  NumInputPorts=2
      settings: SampleTime=tsample  ActiveDisplayYMinimum=-0.16149  ActiveDisplayYMaximum=0.90685
  Selector1 : Selector  InputPortWidth=3  IndexOptions=Index vector (dialog)  Indices=3  OutputSizes=1
  h_hat/h : Scope  Commented=on  NumInputPorts=2
      settings: SampleTime=tsample  ActiveDisplayYMinimum=-0.13002  ActiveDisplayYMaximum=0.15534  DataLoggingVariableName=ScopeData2
  i_out/v_out : Scope  Commented=on  NumInputPorts=2
      settings: SampleTime=tsample  ActiveDisplayYMinimum=-467.6442  ActiveDisplayYMaximum=280.8763  DataLoggingVariableName=ScopeData3
  soc/iout : Scope  Commented=on  NumInputPorts=2
      settings: SampleTime=tsample  ActiveDisplayYMinimum=0.19925  ActiveDisplayYMaximum=0.20008  DataLoggingVariableName=ScopeData4
  wires:
  [icell] -> soc/iout/2
  [vout] -> i_out/v_out/2, Kalman_observer/1(vout(k))
  Selector1/1 -> h_hat/h/1  "h_hat(z)"
  [SOC] -> SOC*/SOC/1, soc/iout/1
  [h] -> h_hat/h/2
  [im] -> i_out/v_out/1  "im+noise"
  Kalman_observer/1(x(k+1|k)) -> Selector1/1
  Kalman_observer/2(SOC) -> SOC*/SOC/2

== system three_level_ttype_pwm/theee-level-inverter-pwm/battery_system/LithiumIonBattery/lithium ion cell analytical ocv ==
  Current Sensor : fl_lib/Electrical/Electrical Sensors/Current Sensor
  PS Constant : fl_lib/Physical Signals/Sources/PS Constant  constant=298.15 K
  PS-Simulink Converter{,1..4} (5 alike) : nesl_utility/PS-Simulink Converter  PhysicalDomain=network_engine_domain  SubClassName=ps_output  LeftPortType=input  RightPortType=output  PseudoPeriodic=off  Frequencies=[]  VectorFormat=1-D array  Unit=inherit  AffineConversion=off
  Voltage Sensor : fl_lib/Electrical/Electrical Sensors/Voltage Sensor
  lithium-ion battery with analytical OCV : lithium_ion_cell_lib/lithium-ion Cell with analytical OCV  Qcell=Q hr*A  N=number_of_cells  E_1=E1 V  E0=E0 V  E1=E1 V  E2=E2 V  E3=E3 V  Elog=Elog V  R0=R0 Ohm  R1=R1 Ohm  C1=C1 F  M=M V  alpha=alpha  u_specify=off  u_priority=High  u=Vdc V  u_nominal_specify=off  u_nominal_unit=V  u_nominal_value=1  u_ocv_specify=off  u_ocv_priority=High  u_ocv=Vdc V  u_ocv_nominal_specify=off  u_ocv_nominal_unit=V  u_ocv_nominal_value=1  icell_specify=off  icell_priority=None  icell=0 A  icell_nominal_specify=off  icell_nominal_unit=A  icell_nominal_value=1  i_r1_specify=off  i_r1_priority=None  i_r1=0 A  i_r1_nominal_specify=off  i_r1_nominal_unit=A  i_r1_nominal_value=1  z_specify=on  z_priority=High  z=soc_init  z_nominal_specify=off  z_nominal_unit=1  z_nominal_value=1  h_specify=off  h_priority=High  h=0  h_nominal_specify=off  h_nominal_unit=1  h_nominal_value=1
      settings: InternalSimscapePortConfiguration="{\"Bottom\":[],\"Left\":[{\"id\":\"T\",\"label\":\"T\",\"type\":\"input\"}],\"Right\":[{\"id\":\"u_p\",\"label\":\"u+\",\"type\":\"foundation.electrical.electrical\"},{\"id\":\"u_n\",\"label\":\"u-\",\"type\":\"foundation.electrical.electrical\"},{\"id\":\"z_out\",\"label\":\"SOC\",\"type\":\"output\"},{\"id\":\"i_r1_out\",\"label\":\"i_r1\",\"type\":\"output\"},{\"id\":\"h_out\",\"label\":\"hysteresis\",\"type\":\"output\"}],\"Top\":[]}"
  white_noise : Subsystem
  U+ : PMIOPort  Side=Right
  U- : PMIOPort  Port=2  Side=Right
  tag scope: SOC=global, h=global, icell=global, im=global, vout=global
  wires:
  PS-Simulink Converter3/1 -> [SOC]  "SOC*"
  PS-Simulink Converter2/1 -> [icell]  "icell"
  PS-Simulink Converter4/1 -> [h]  "h(t)"
  white_noise/1(out) -> [im]
  PS-Simulink Converter1/1 -> white_noise/1(in)  "i(k)"
  PS-Simulink Converter/1 -> [vout]  "vout(k)"
  connections:
  lithium-ion battery with analytical OCV/RConn5 -- PS-Simulink Converter4/LConn1
  lithium-ion battery with analytical OCV/RConn4 -- PS-Simulink Converter2/LConn1
  lithium-ion battery with analytical OCV/RConn3 -- PS-Simulink Converter3/LConn1
  lithium-ion battery with analytical OCV/RConn1 -- Current Sensor/LConn1
  Current Sensor/RConn1 -- PS-Simulink Converter1/LConn1
  lithium-ion battery with analytical OCV/RConn2 -- U-/RConn1 -- Voltage Sensor/RConn2
  U+/RConn1 -- Voltage Sensor/LConn1 -- Current Sensor/RConn2
  PS-Simulink Converter/LConn1 -- Voltage Sensor/RConn1
  lithium-ion battery with analytical OCV/LConn1 -- PS Constant/RConn1

== system three_level_ttype_pwm/theee-level-inverter-pwm/pwm_commands/PWM generator u/carry_n ==
  phase : Inport
  Clock : Clock
  Constant2 : Constant  Value=1/f
  Constant4 : Constant  Value=-1
  Gain4 : Gain  Gain=1/2
  Gain5 : Gain  Gain=1/(pi/2)
  MATLAB Function : MATLAB Function  TreatAsAtomicUnit=on
  Sum3 : Sum  Inputs=|++
  trn : Outport
  wires:
  phase/1 -> MATLAB Function/2(phase)
  Clock/1 -> MATLAB Function/1(t)
  Constant4/1 -> Sum3/2
  MATLAB Function/1(y) -> Gain5/1
  Sum3/1 -> Gain4/1
  Constant2/1 -> MATLAB Function/3(period)
  Gain4/1 -> trn/1
  Gain5/1 -> Sum3/1

== system three_level_ttype_pwm/theee-level-inverter-pwm/pwm_commands/PWM generator u/carry_p ==
  phase : Inport
  Clock : Clock
  Constant2 : Constant  Value=1/f
  Constant4 : Constant
  Gain4 : Gain  Gain=1/2
  Gain5 : Gain  Gain=1/(pi/2)
  MATLAB Function : MATLAB Function  TreatAsAtomicUnit=on
  Sum3 : Sum  Inputs=|++
  trp : Outport
  wires:
  Gain5/1 -> Sum3/1
  Gain4/1 -> trp/1
  Constant2/1 -> MATLAB Function/3(period)
  Sum3/1 -> Gain4/1
  MATLAB Function/1(y) -> Gain5/1
  Constant4/1 -> Sum3/2
  Clock/1 -> MATLAB Function/1(t)
  phase/1 -> MATLAB Function/2(phase)

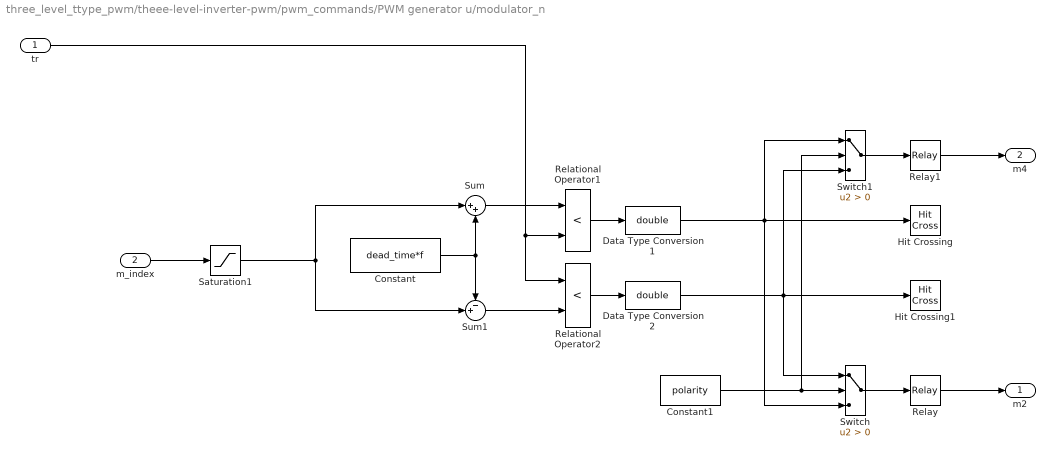
== system three_level_ttype_pwm/theee-level-inverter-pwm/pwm_commands/PWM generator u/modulator_n ==
  tr : Inport
  m_index : Inport  Port=2
  Constant : Constant  Value=dead_time*f
  Constant1 : Constant  Value=polarity
  Data Type Conversion1 : DataTypeConversion  OutDataTypeStr=double
  Data Type Conversion2 : DataTypeConversion  OutDataTypeStr=double
  Hit Crossing : HitCross  ShowOutputPort=off
  Hit Crossing1 : HitCross  ShowOutputPort=off
  Relational Operator1 : RelationalOperator  Operator=<  InputSameDT=off
  Relational Operator2 : RelationalOperator  Operator=<  InputSameDT=off
  Relay : Relay  OnOutputValue=pos_cmd_gate  OffOutputValue=neg_cmd_gate
  Relay1 : Relay  OnOutputValue=pos_cmd_gate  OffOutputValue=neg_cmd_gate
  Saturation1 : Saturate  UpperLimit=m_up  LowerLimit=m_low
  Sum : Sum  Inputs=|++  SaturateOnIntegerOverflow=on
  Sum1 : Sum  Inputs=-+|  SaturateOnIntegerOverflow=on
  Switch : Switch  Criteria=u2 > Threshold  SaturateOnIntegerOverflow=off  InputSameDT=off
  Switch1 : Switch  Criteria=u2 > Threshold  SaturateOnIntegerOverflow=off  InputSameDT=off
  m2 : Outport
  m4 : Outport  Port=2
  wires:
  Switch1/1 -> Relay1/1
  tr/1 -> Relational Operator1/2, Relational Operator2/1
  Sum/1 -> Relational Operator1/1
  Constant/1 -> Sum1/1, Sum/2
  Switch/1 -> Relay/1
  Data Type Conversion2/1 -> Hit Crossing1/1, Switch1/3, Switch/1
  Constant1/1 -> Switch/2, Switch1/2
  Saturation1/1 -> Sum1/2, Sum/1
  Sum1/1 -> Relational Operator2/2
  Data Type Conversion1/1 -> Switch1/1, Switch/3, Hit Crossing/1
  Relational Operator1/1 -> Data Type Conversion1/1
  Relational Operator2/1 -> Data Type Conversion2/1
  m_index/1 -> Saturation1/1
  Relay/1 -> m2/1
  Relay1/1 -> m4/1

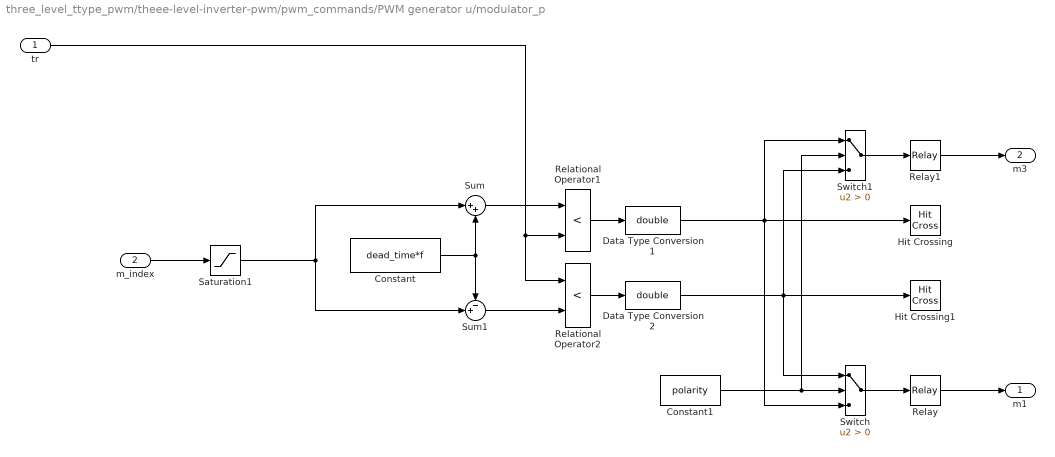
== system three_level_ttype_pwm/theee-level-inverter-pwm/pwm_commands/PWM generator u/modulator_p ==
  tr : Inport
  m_index : Inport  Port=2
  Constant : Constant  Value=dead_time*f
  Constant1 : Constant  Value=polarity
  Data Type Conversion1 : DataTypeConversion  OutDataTypeStr=double
  Data Type Conversion2 : DataTypeConversion  OutDataTypeStr=double
  Hit Crossing : HitCross  ShowOutputPort=off
  Hit Crossing1 : HitCross  ShowOutputPort=off
  Relational Operator1 : RelationalOperator  Operator=<  InputSameDT=off
  Relational Operator2 : RelationalOperator  Operator=<  InputSameDT=off
  Relay : Relay  OnOutputValue=pos_cmd_gate  OffOutputValue=neg_cmd_gate
  Relay1 : Relay  OnOutputValue=pos_cmd_gate  OffOutputValue=neg_cmd_gate
  Saturation1 : Saturate  UpperLimit=m_up  LowerLimit=m_low
  Sum : Sum  Inputs=|++  SaturateOnIntegerOverflow=on
  Sum1 : Sum  Inputs=-+|  SaturateOnIntegerOverflow=on
  Switch : Switch  Criteria=u2 > Threshold  SaturateOnIntegerOverflow=off  InputSameDT=off
  Switch1 : Switch  Criteria=u2 > Threshold  SaturateOnIntegerOverflow=off  InputSameDT=off
  m1 : Outport
  m3 : Outport  Port=2
  wires:
  m_index/1 -> Saturation1/1
  Relational Operator2/1 -> Data Type Conversion2/1
  Relational Operator1/1 -> Data Type Conversion1/1
  Data Type Conversion1/1 -> Hit Crossing/1, Switch/3, Switch1/1
  Sum1/1 -> Relational Operator2/2
  Saturation1/1 -> Sum/1, Sum1/2
  Constant1/1 -> Switch1/2, Switch/2
  Data Type Conversion2/1 -> Switch/1, Switch1/3, Hit Crossing1/1
  Switch/1 -> Relay/1
  Constant/1 -> Sum/2, Sum1/1
  Sum/1 -> Relational Operator1/1
  tr/1 -> Relational Operator2/1, Relational Operator1/2
  Switch1/1 -> Relay1/1
  Relay/1 -> m1/1
  Relay1/1 -> m3/1

== system three_level_ttype_pwm/theee-level-inverter-pwm/pwm_commands/PWM generator v/carry_n ==
  phase : Inport
  Clock : Clock
  Constant2 : Constant  Value=1/f
  Constant4 : Constant  Value=-1
  Gain4 : Gain  Gain=1/2
  Gain5 : Gain  Gain=1/(pi/2)
  MATLAB Function : MATLAB Function  TreatAsAtomicUnit=on
  Sum3 : Sum  Inputs=|++
  trn : Outport
  wires:
  Gain5/1 -> Sum3/1
  Gain4/1 -> trn/1
  Constant2/1 -> MATLAB Function/3(period)
  Sum3/1 -> Gain4/1
  MATLAB Function/1(y) -> Gain5/1
  Constant4/1 -> Sum3/2
  Clock/1 -> MATLAB Function/1(t)
  phase/1 -> MATLAB Function/2(phase)

== system three_level_ttype_pwm/theee-level-inverter-pwm/pwm_commands/PWM generator v/carry_p ==
  phase : Inport
  Clock : Clock
  Constant2 : Constant  Value=1/f
  Constant4 : Constant
  Gain4 : Gain  Gain=1/2
  Gain5 : Gain  Gain=1/(pi/2)
  MATLAB Function : MATLAB Function  TreatAsAtomicUnit=on
  Sum3 : Sum  Inputs=|++
  trp : Outport
  wires:
  phase/1 -> MATLAB Function/2(phase)
  Clock/1 -> MATLAB Function/1(t)
  Constant4/1 -> Sum3/2
  MATLAB Function/1(y) -> Gain5/1
  Sum3/1 -> Gain4/1
  Constant2/1 -> MATLAB Function/3(period)
  Gain4/1 -> trp/1
  Gain5/1 -> Sum3/1

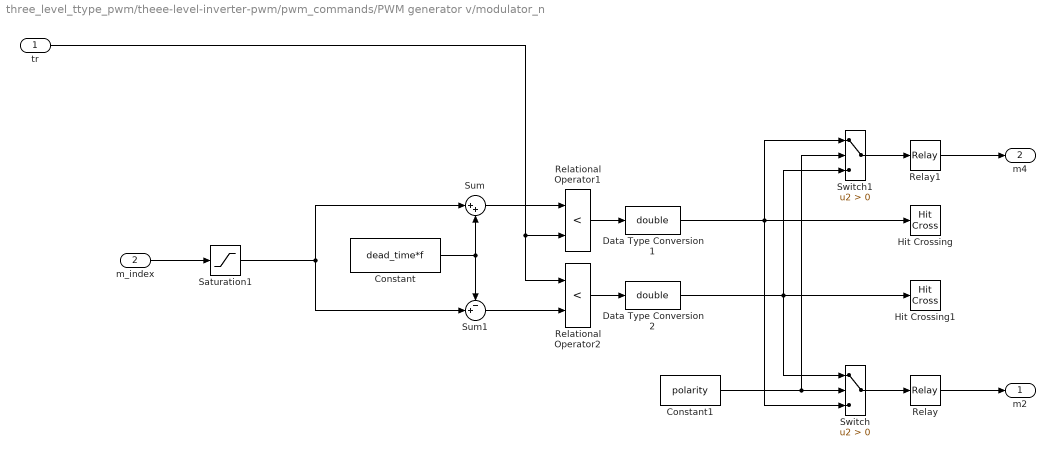
== system three_level_ttype_pwm/theee-level-inverter-pwm/pwm_commands/PWM generator v/modulator_n ==
  tr : Inport
  m_index : Inport  Port=2
  Constant : Constant  Value=dead_time*f
  Constant1 : Constant  Value=polarity
  Data Type Conversion1 : DataTypeConversion  OutDataTypeStr=double
  Data Type Conversion2 : DataTypeConversion  OutDataTypeStr=double
  Hit Crossing : HitCross  ShowOutputPort=off
  Hit Crossing1 : HitCross  ShowOutputPort=off
  Relational Operator1 : RelationalOperator  Operator=<  InputSameDT=off
  Relational Operator2 : RelationalOperator  Operator=<  InputSameDT=off
  Relay : Relay  OnOutputValue=pos_cmd_gate  OffOutputValue=neg_cmd_gate
  Relay1 : Relay  OnOutputValue=pos_cmd_gate  OffOutputValue=neg_cmd_gate
  Saturation1 : Saturate  UpperLimit=m_up  LowerLimit=m_low
  Sum : Sum  Inputs=|++  SaturateOnIntegerOverflow=on
  Sum1 : Sum  Inputs=-+|  SaturateOnIntegerOverflow=on
  Switch : Switch  Criteria=u2 > Threshold  SaturateOnIntegerOverflow=off  InputSameDT=off
  Switch1 : Switch  Criteria=u2 > Threshold  SaturateOnIntegerOverflow=off  InputSameDT=off
  m2 : Outport
  m4 : Outport  Port=2
  wires:
  Relay1/1 -> m4/1
  Relay/1 -> m2/1
  m_index/1 -> Saturation1/1
  Relational Operator2/1 -> Data Type Conversion2/1
  Relational Operator1/1 -> Data Type Conversion1/1
  Data Type Conversion1/1 -> Hit Crossing/1, Switch/3, Switch1/1
  Sum1/1 -> Relational Operator2/2
  Saturation1/1 -> Sum/1, Sum1/2
  Constant1/1 -> Switch1/2, Switch/2
  Data Type Conversion2/1 -> Switch/1, Switch1/3, Hit Crossing1/1
  Switch/1 -> Relay/1
  Constant/1 -> Sum/2, Sum1/1
  Sum/1 -> Relational Operator1/1
  tr/1 -> Relational Operator2/1, Relational Operator1/2
  Switch1/1 -> Relay1/1

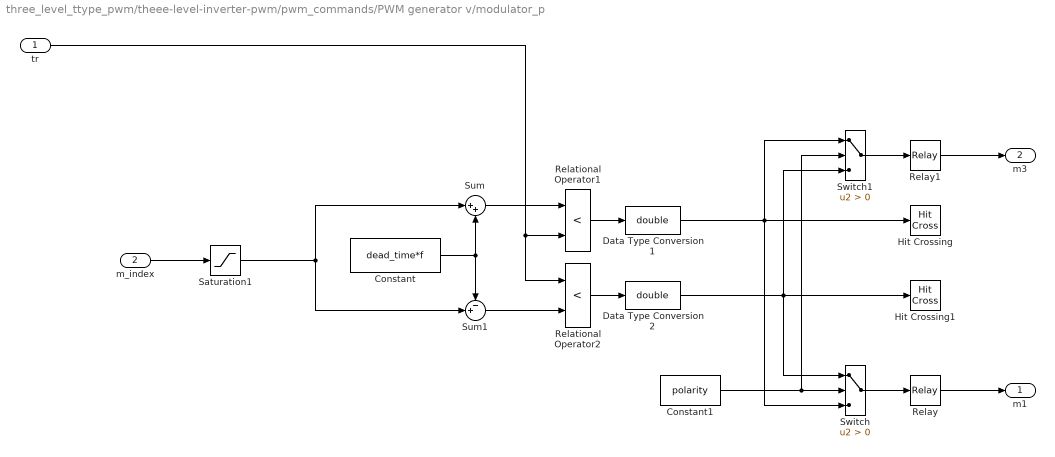
== system three_level_ttype_pwm/theee-level-inverter-pwm/pwm_commands/PWM generator v/modulator_p ==
  tr : Inport
  m_index : Inport  Port=2
  Constant : Constant  Value=dead_time*f
  Constant1 : Constant  Value=polarity
  Data Type Conversion1 : DataTypeConversion  OutDataTypeStr=double
  Data Type Conversion2 : DataTypeConversion  OutDataTypeStr=double
  Hit Crossing : HitCross  ShowOutputPort=off
  Hit Crossing1 : HitCross  ShowOutputPort=off
  Relational Operator1 : RelationalOperator  Operator=<  InputSameDT=off
  Relational Operator2 : RelationalOperator  Operator=<  InputSameDT=off
  Relay : Relay  OnOutputValue=pos_cmd_gate  OffOutputValue=neg_cmd_gate
  Relay1 : Relay  OnOutputValue=pos_cmd_gate  OffOutputValue=neg_cmd_gate
  Saturation1 : Saturate  UpperLimit=m_up  LowerLimit=m_low
  Sum : Sum  Inputs=|++  SaturateOnIntegerOverflow=on
  Sum1 : Sum  Inputs=-+|  SaturateOnIntegerOverflow=on
  Switch : Switch  Criteria=u2 > Threshold  SaturateOnIntegerOverflow=off  InputSameDT=off
  Switch1 : Switch  Criteria=u2 > Threshold  SaturateOnIntegerOverflow=off  InputSameDT=off
  m1 : Outport
  m3 : Outport  Port=2
  wires:
  Relay1/1 -> m3/1
  Relay/1 -> m1/1
  Switch1/1 -> Relay1/1
  tr/1 -> Relational Operator1/2, Relational Operator2/1
  Sum/1 -> Relational Operator1/1
  Constant/1 -> Sum1/1, Sum/2
  Switch/1 -> Relay/1
  Data Type Conversion2/1 -> Hit Crossing1/1, Switch1/3, Switch/1
  Constant1/1 -> Switch/2, Switch1/2
  Saturation1/1 -> Sum1/2, Sum/1
  Sum1/1 -> Relational Operator2/2
  Data Type Conversion1/1 -> Switch1/1, Switch/3, Hit Crossing/1
  Relational Operator1/1 -> Data Type Conversion1/1
  Relational Operator2/1 -> Data Type Conversion2/1
  m_index/1 -> Saturation1/1

== system three_level_ttype_pwm/theee-level-inverter-pwm/pwm_commands/PWM generator v1/carry_n ==
  phase : Inport
  Clock : Clock
  Constant2 : Constant  Value=1/f
  Constant4 : Constant  Value=-1
  Gain4 : Gain  Gain=1/2
  Gain5 : Gain  Gain=1/(pi/2)
  MATLAB Function : MATLAB Function  TreatAsAtomicUnit=on
  Sum3 : Sum  Inputs=|++
  trn : Outport
  wires:
  phase/1 -> MATLAB Function/2(phase)
  Clock/1 -> MATLAB Function/1(t)
  Constant4/1 -> Sum3/2
  MATLAB Function/1(y) -> Gain5/1
  Sum3/1 -> Gain4/1
  Constant2/1 -> MATLAB Function/3(period)
  Gain4/1 -> trn/1
  Gain5/1 -> Sum3/1

== system three_level_ttype_pwm/theee-level-inverter-pwm/pwm_commands/PWM generator v1/carry_p ==
  phase : Inport
  Clock : Clock
  Constant2 : Constant  Value=1/f
  Constant4 : Constant
  Gain4 : Gain  Gain=1/2
  Gain5 : Gain  Gain=1/(pi/2)
  MATLAB Function : MATLAB Function  TreatAsAtomicUnit=on
  Sum3 : Sum  Inputs=|++
  trp : Outport
  wires:
  Gain5/1 -> Sum3/1
  Gain4/1 -> trp/1
  Constant2/1 -> MATLAB Function/3(period)
  Sum3/1 -> Gain4/1
  MATLAB Function/1(y) -> Gain5/1
  Constant4/1 -> Sum3/2
  Clock/1 -> MATLAB Function/1(t)
  phase/1 -> MATLAB Function/2(phase)

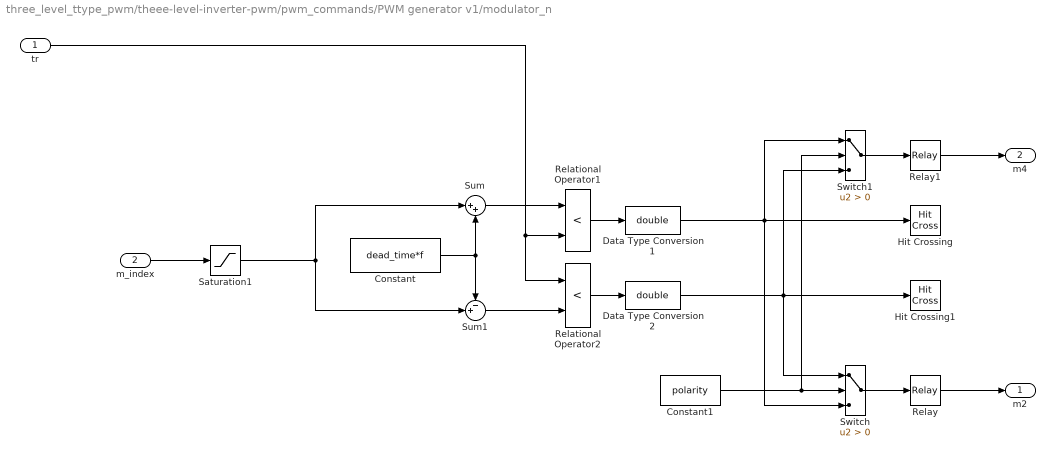
== system three_level_ttype_pwm/theee-level-inverter-pwm/pwm_commands/PWM generator v1/modulator_n ==
  tr : Inport
  m_index : Inport  Port=2
  Constant : Constant  Value=dead_time*f
  Constant1 : Constant  Value=polarity
  Data Type Conversion1 : DataTypeConversion  OutDataTypeStr=double
  Data Type Conversion2 : DataTypeConversion  OutDataTypeStr=double
  Hit Crossing : HitCross  ShowOutputPort=off
  Hit Crossing1 : HitCross  ShowOutputPort=off
  Relational Operator1 : RelationalOperator  Operator=<  InputSameDT=off
  Relational Operator2 : RelationalOperator  Operator=<  InputSameDT=off
  Relay : Relay  OnOutputValue=pos_cmd_gate  OffOutputValue=neg_cmd_gate
  Relay1 : Relay  OnOutputValue=pos_cmd_gate  OffOutputValue=neg_cmd_gate
  Saturation1 : Saturate  UpperLimit=m_up  LowerLimit=m_low
  Sum : Sum  Inputs=|++  SaturateOnIntegerOverflow=on
  Sum1 : Sum  Inputs=-+|  SaturateOnIntegerOverflow=on
  Switch : Switch  Criteria=u2 > Threshold  SaturateOnIntegerOverflow=off  InputSameDT=off
  Switch1 : Switch  Criteria=u2 > Threshold  SaturateOnIntegerOverflow=off  InputSameDT=off
  m2 : Outport
  m4 : Outport  Port=2
  wires:
  Switch1/1 -> Relay1/1
  tr/1 -> Relational Operator1/2, Relational Operator2/1
  Sum/1 -> Relational Operator1/1
  Constant/1 -> Sum1/1, Sum/2
  Switch/1 -> Relay/1
  Data Type Conversion2/1 -> Hit Crossing1/1, Switch1/3, Switch/1
  Constant1/1 -> Switch/2, Switch1/2
  Saturation1/1 -> Sum1/2, Sum/1
  Sum1/1 -> Relational Operator2/2
  Data Type Conversion1/1 -> Switch1/1, Switch/3, Hit Crossing/1
  Relational Operator1/1 -> Data Type Conversion1/1
  Relational Operator2/1 -> Data Type Conversion2/1
  m_index/1 -> Saturation1/1
  Relay/1 -> m2/1
  Relay1/1 -> m4/1

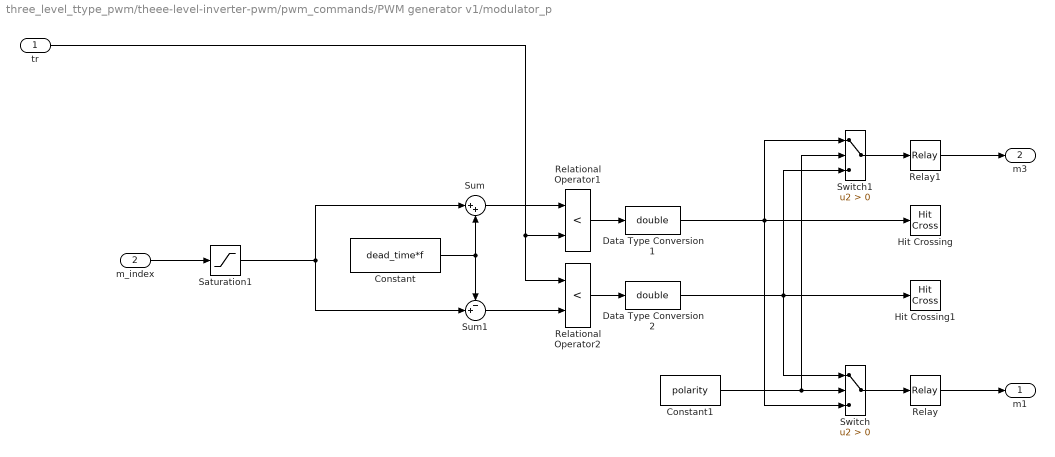
== system three_level_ttype_pwm/theee-level-inverter-pwm/pwm_commands/PWM generator v1/modulator_p ==
  tr : Inport
  m_index : Inport  Port=2
  Constant : Constant  Value=dead_time*f
  Constant1 : Constant  Value=polarity
  Data Type Conversion1 : DataTypeConversion  OutDataTypeStr=double
  Data Type Conversion2 : DataTypeConversion  OutDataTypeStr=double
  Hit Crossing : HitCross  ShowOutputPort=off
  Hit Crossing1 : HitCross  ShowOutputPort=off
  Relational Operator1 : RelationalOperator  Operator=<  InputSameDT=off
  Relational Operator2 : RelationalOperator  Operator=<  InputSameDT=off
  Relay : Relay  OnOutputValue=pos_cmd_gate  OffOutputValue=neg_cmd_gate
  Relay1 : Relay  OnOutputValue=pos_cmd_gate  OffOutputValue=neg_cmd_gate
  Saturation1 : Saturate  UpperLimit=m_up  LowerLimit=m_low
  Sum : Sum  Inputs=|++  SaturateOnIntegerOverflow=on
  Sum1 : Sum  Inputs=-+|  SaturateOnIntegerOverflow=on
  Switch : Switch  Criteria=u2 > Threshold  SaturateOnIntegerOverflow=off  InputSameDT=off
  Switch1 : Switch  Criteria=u2 > Threshold  SaturateOnIntegerOverflow=off  InputSameDT=off
  m1 : Outport
  m3 : Outport  Port=2
  wires:
  m_index/1 -> Saturation1/1
  Relational Operator2/1 -> Data Type Conversion2/1
  Relational Operator1/1 -> Data Type Conversion1/1
  Data Type Conversion1/1 -> Hit Crossing/1, Switch/3, Switch1/1
  Sum1/1 -> Relational Operator2/2
  Saturation1/1 -> Sum/1, Sum1/2
  Constant1/1 -> Switch1/2, Switch/2
  Data Type Conversion2/1 -> Switch/1, Switch1/3, Hit Crossing1/1
  Switch/1 -> Relay/1
  Constant/1 -> Sum/2, Sum1/1
  Sum/1 -> Relational Operator1/1
  tr/1 -> Relational Operator2/1, Relational Operator1/2
  Switch1/1 -> Relay1/1
  Relay/1 -> m1/1
  Relay1/1 -> m3/1
